simulink model "m20150807_motor28335_21"  (R2012b)
settings: Solver=FixedStepDiscrete  StartTime=0.0  StopTime=5  FixedStep=5e-5  RelTol=1e-3
PostLoadFcn:
  | c2000demoscallback(1);
  | Ts = 50e-6;
model workspace (MAT data in the model file):
  polePairs = 4
  encoderResolution = 2500
  indexOffset = 0
undefined symbols (not defined in the file or in its folder): Down, Up
libraries: c2833xlib x13, c28xdmclib x10, tiiqmathlib x8, simulink x4, c280xlib x4, idelinklib_common x4, c2000_demo_controls x1, idelinklib_tgtpref x1
settings Model: FPTRunName=Active  Creator=The MathWorks Inc.  LastModifiedBy=Krunal
settings DataIOCC: SignalLoggingSaveFormat=ModelDataLogs  SaveOutput=off  SaveTime=off
settings OptimizationCC: InlineParams=on  InlineInvariantSignals=on  InitFltsAndDblsToZero=on  NoFixptDivByZeroProtection=on  EfficientFloat2IntCast=on  EfficientMapNaN2IntZero=off  OptimizeModelRefInitCode=on
settings DebuggingCC: SignalResolutionControl=TryResolveAllWithWarning  InheritedTsInSrcMsg=none  MultiTaskDSMMsg=warning  MultiTaskCondExecSysMsg=none  SigSpecEnsureSampleTimeMsg=none  IntegerOverflowMsg=none  ParameterPrecisionLossMsg=none  FcnCallInpInsideContextMsg=UseLocalSettings  StrictBusMsg=None
settings HardwareCC: ProdBitPerChar=16  ProdBitPerInt=16  ProdBitPerPointer=16  ProdLargestAtomicInteger=Integer  ProdIntDivRoundTo=Zero  ProdEndianess=LittleEndian  ProdWordSize=16  ProdHWDeviceType=Texas Instruments->C2000  TargetBitPerChar=16  TargetBitPerInt=16  TargetBitPerPointer=16  TargetIntDivRoundTo=Zero  TargetEndianess=LittleEndian  TargetWordSize=16  TargetHWDeviceType=TI C2000
settings RTWCC: SystemTargetFile=idelink_ert.tlc  TLCOptions="-aCustomTestInterfaceFile=\"pil_gen_interface.tlc\""  GenerateMakefile=off  TemplateMakefile=none  Description=IDE Link ERT  ProcessScript=ccslink_ert_make_rtw_hook
settings CodeAppCC: IgnoreCustomStorageClasses=off
settings ConfigurationSet: Description=SimMechanics 2G

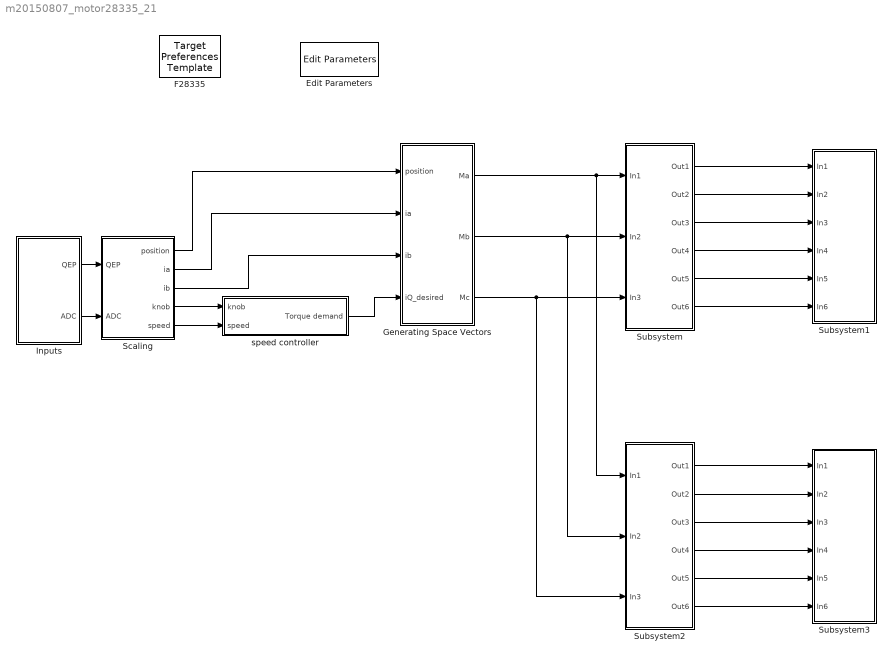
== system m20150807_motor28335_21 ==
  Edit Parameters : c2000_demo_controls/Edit Parameters  Priority=4  polePairs=4  encoderResolution=2500  IndexOffset=0
  F28335 : idelinklib_tgtpref/Target Preferences Template  Tag=ccslinktgtpref_ccsv5  library=off
  Generating Space Vectors : Subsystem
  Inputs : Subsystem
  Scaling : Subsystem
  Subsystem : Subsystem
  Subsystem1 : Subsystem
  Subsystem2 : Subsystem
  Subsystem3 : Subsystem
  speed controller : Subsystem
  wires:
  Scaling/1(position) -> Generating Space Vectors/1(position)
  Scaling/2(ia) -> Generating Space Vectors/2(ia)
  Scaling/3(ib) -> Generating Space Vectors/3(ib)
  Scaling/4(knob) -> speed controller/1(knob)
  Inputs/2(ADC) -> Scaling/2(ADC)
  speed controller/1(Torque demand) -> Generating Space Vectors/4(iQ_desired)
  Scaling/5(speed) -> speed controller/2(speed)
  Inputs/1(QEP) -> Scaling/1(QEP)
  Subsystem/1(Out1) -> Subsystem1/1(In1)
  Subsystem/2(Out2) -> Subsystem1/2(In2)
  Subsystem/3(Out3) -> Subsystem1/3(In3)
  Subsystem/4(Out4) -> Subsystem1/4(In4)
  Subsystem/5(Out5) -> Subsystem1/5(In5)
  Subsystem/6(Out6) -> Subsystem1/6(In6)
  Generating Space Vectors/1(Ma) -> Subsystem2/1(In1), Subsystem/1(In1)
  Generating Space Vectors/2(Mb) -> Subsystem2/2(In2), Subsystem/2(In2)
  Generating Space Vectors/3(Mc) -> Subsystem2/3(In3), Subsystem/3(In3)
  Subsystem2/1(Out1) -> Subsystem3/1(In1)
  Subsystem2/2(Out2) -> Subsystem3/2(In2)
  Subsystem2/3(Out3) -> Subsystem3/3(In3)
  Subsystem2/4(Out4) -> Subsystem3/4(In4)
  Subsystem2/5(Out5) -> Subsystem3/5(In5)
  Subsystem2/6(Out6) -> Subsystem3/6(In6)

== system m20150807_motor28335_21/Generating Space Vectors ==
  position : Inport
  ia : Inport  Port=2
  ib : Inport  Port=3
  iQ_desired : Inport  Port=4
  Generating Raw Space Vectors : Subsystem
  Rate Transition2 : RateTransition  Integrity=off
  Ma : Outport
  Mb : Outport  Port=2
  Mc : Outport  Port=3
  wires:
  ia/1 -> Generating Raw Space Vectors/1(Ia)
  ib/1 -> Generating Raw Space Vectors/2(Ib)
  position/1 -> Generating Raw Space Vectors/3(position)
  Generating Raw Space Vectors/1(Out1) -> Ma/1
  Generating Raw Space Vectors/2(Out2) -> Mb/1
  Generating Raw Space Vectors/3(Out3) -> Mc/1
  iQ_desired/1 -> Rate Transition2/1
  Rate Transition2/1 -> Generating Raw Space Vectors/4(iQ_desired)

== system m20150807_motor28335_21/Inputs ==
  note: Hardware Inputs
  ADC1 : c280xlib/ADC  useModule=A  useMode=Sequential  sourceSOC=Software  sourceSOC1=Software  sourceSOC2=ePWMxB  xint2_ADCSOC=31  Ts=Ts  dType=uint16  postInterrupt=off  numConversionsSingle=3  numConversionsDouble=1  conv0=ADCINA0  conv1=ADCINA1  conv2=ADCINA2  conv3=ADCINA3  conv4=ADCINA4  conv5=ADCINA5  conv6=ADCINA6  conv7=ADCINA7  conv8=ADCINB0  conv9=ADCINB1  conv10=ADCINB2  conv11=ADCINB3  conv12=ADCINB4  conv13=ADCINB5  conv14=ADCINB6  conv15=ADCINB7  convAB0=ADCINA0 and ADCINB0  convAB1=ADCINA1 and ADCINB1  convAB2=ADCINA2 and ADCINB2  convAB3=ADCINA3 and ADCINB3  convAB4=ADCINA4 and ADCINB4  convAB5=ADCINA5 and ADCINB5  convAB6=ADCINA6 and ADCINB6  convAB7=ADCINA7 and ADCINB7  convA0=ADCINA0  convA1=ADCINA1  convA2=ADCINA7  convA3=ADCINA3  convA4=ADCINA4  convA5=ADCINA5  convA6=ADCINA6  convA7=ADCINA7  convB0=ADCINB0  convB1=ADCINB1  convB2=ADCINB2  convB3=ADCINB3  convB4=ADCINB4  convB5=ADCINB5  convB6=ADCINB6  convB7=ADCINB7  c28xmultiPort=off  endma=off  chdma=1
  eQEP : c280xlib/eQEP  useModule=eQEP1  pcInputmode=Quadrature-count  externalClockrate=2x resolution: Count the rising/falling edge  swapPolarityselection=Clockwise  qdfOutputport=off  qapPolarityselection=off  qbpPolarityselection=off  qipPolarityselection=off  qspPolarityselection=off  igatePolarityselection=off  sampleTime=Ts  pcOutputport=on  pcMaximumvalue=65535  indexInitializationcheck=off  indexInitializationevent=Rising edge  strobeInitializationcheck=off  strobeInitializationevent=Rising edge  softwareInitializationcheck=off  softwareInitializationsource=Set to init value at start up  softwareInitializationmode=on  pcInitialvalue=2147483648  pcResetmode=Reset on an index event  ieloutputport=off  indexEventlatch=Rising edge  seloutputport=off  strobeEventlatch=Rising edge  pcefOutputport=off  enableEqepcapture=off  qctmrOutputport=off  qcprdOutputport=off  captureTimerprescaler=128  upEventprescaler=128  overflowErrorflag=off  directionErrorflag=off  captureTimerposition=On position counter read  unitTimerperiod=100000000  captureTimerlatch=off  capturePeriodlatch=off  positionCounterlatch=off  soenPolarityselection=off  spselPolarityselection=Index pin is used for sync output  compareValuesource=Specify via dialog  shadowMode=Load on QPOSCNT=0  compareValue=4294967295  syncOutputwidth=1  polaritySyncoutput=Active high  watchdogEnable=off  watchdogTimer=65535  outport1Datatype=auto  outport2Datatype=auto  outport3Datatype=auto  outport4Datatype=auto  outport5Datatype=auto  outport6Datatype=auto  outport7Datatype=auto  outport8Datatype=auto  outport9Datatype=auto  outport10Datatype=auto  outport11Datatype=auto  outport12Datatype=auto  eqepinterrupt_pce=off  eqepinterrupt_qpe=off  eqepinterrupt_qdc=off  eqepinterrupt_wto=off  eqepinterrupt_pcu=off  eqepinterrupt_pco=off  eqepinterrupt_pcr=off  eqepinterrupt_pcm=off  eqepinterrupt_sel=off  eqepinterrupt_iel=off  eqepinterrupt_uto=off  pheOutputport=off  watchdogOutputport=off  outport13Datatype=auto  outport14Datatype=auto
  QEP : Outport
  ADC : Outport  Port=2
  wires:
  eQEP/1 -> QEP/1
  ADC1/1 -> ADC/1

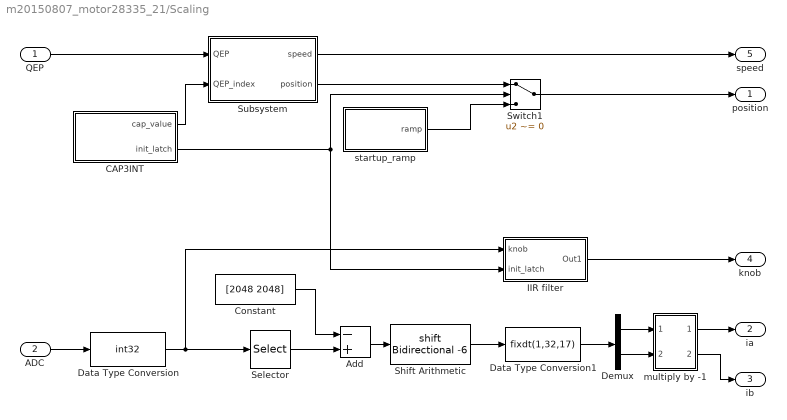
== system m20150807_motor28335_21/Scaling ==
  QEP : Inport
  ADC : Inport  Port=2
  Add : Sum  Inputs=-+
  CAP3INT : Subsystem
  Constant : Constant  Value=[2048 2048]  OutDataTypeStr=int32
  Data Type Conversion : DataTypeConversion  OutDataTypeStr=int32  ConvertRealWorld=Stored Integer (SI)
  Data Type Conversion1 : DataTypeConversion  OutDataTypeStr=fixdt(1,32,17)  ConvertRealWorld=Stored Integer (SI)
  Demux : Demux  Outputs=2
  IIR filter : Subsystem
  Selector : Selector  InputPortWidth=3  IndexOptions=Index vector (dialog)  Indices=[1 2]  OutputSizes=1
  Shift Arithmetic : ArithShift  BitShiftNumber=-6
  Subsystem : Subsystem
  Switch1 : Switch  Criteria=u2 ~= 0
  multiply by -1 : Subsystem
  startup_ramp : Subsystem
  position : Outport
  ia : Outport  Port=2
  ib : Outport  Port=3
  knob : Outport  Port=4
  speed : Outport  Port=5
  wires:
  CAP3INT/1(cap_value) -> Subsystem/2(QEP_index)
  CAP3INT/2(init_latch) -> Switch1/2, IIR filter/2(init_latch)
  startup_ramp/1(ramp) -> Switch1/3
  Subsystem/2(position) -> Switch1/1
  Data Type Conversion/1 -> Selector/1, IIR filter/1(knob)
  IIR filter/1(Out1) -> knob/1
  Constant/1 -> Add/1
  Selector/1 -> Add/2
  Add/1 -> Shift Arithmetic/1
  Shift Arithmetic/1 -> Data Type Conversion1/1
  Data Type Conversion1/1 -> Demux/1
  Demux/1 -> multiply by -1/1(In1)
  Demux/2 -> multiply by -1/2(In2)
  multiply by -1/1(Out1) -> ia/1
  multiply by -1/2(Out2) -> ib/1
  QEP/1 -> Subsystem/1(QEP)
  ADC/1 -> Data Type Conversion/1
  Switch1/1 -> position/1
  Subsystem/1(speed) -> speed/1

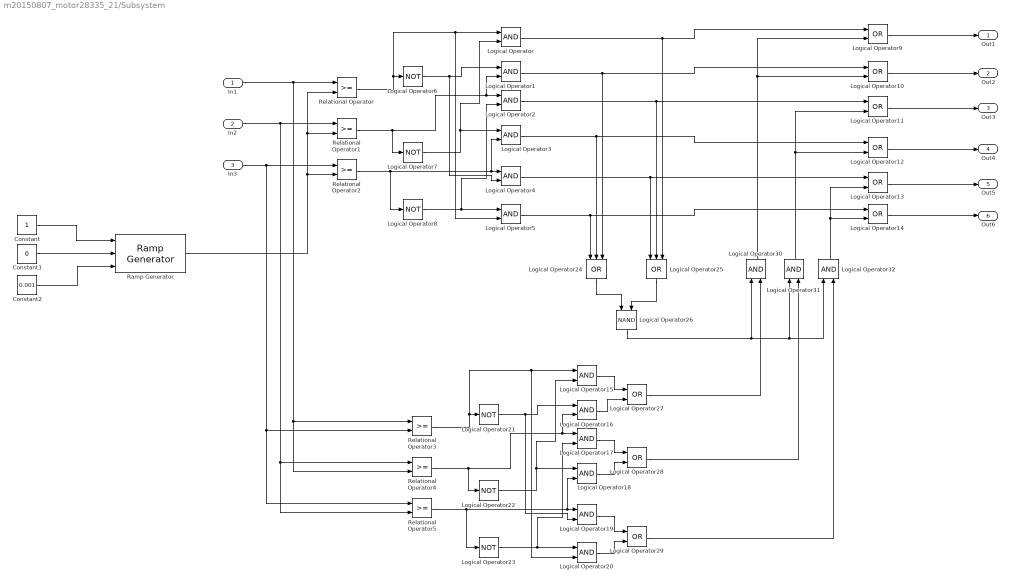
== system m20150807_motor28335_21/Subsystem ==
  In1 : Inport
  In2 : Inport  Port=2
  In3 : Inport  Port=3
  Constant : Constant  OutDataTypeStr=fixdt(1,32,2^-9,0)  SampleTime=0.001
  Constant1 : Constant  Value=0  OutDataTypeStr=fixdt(1,32,2^-9,0)
  Constant2 : Constant  Value=0.001  OutDataTypeStr=fixdt(1,32,2^-9,0)
  Logical Operator{,1..5,15..20,30..32} (15 alike) : Logic  AllPortsSameDT=off  OutDataTypeStr=boolean
  Logical Operator{9..14,27..29} (9 alike) : Logic  Operator=OR  AllPortsSameDT=off  OutDataTypeStr=boolean
  Logical Operator{6..8,21..23} (6 alike) : Logic  Operator=NOT  AllPortsSameDT=off  OutDataTypeStr=boolean
  Logical Operator24 : Logic  Operator=OR  Inputs=3  AllPortsSameDT=off  OutDataTypeStr=boolean
  Logical Operator25 : Logic  Operator=OR  Inputs=3  AllPortsSameDT=off  OutDataTypeStr=boolean
  Logical Operator26 : Logic  Operator=NAND  AllPortsSameDT=off  OutDataTypeStr=boolean
  Ramp Generator : c28xdmclib/Ramp Generator  step_angle_max=1
  Relational Operator{,1..5} (6 alike) : RelationalOperator  OutDataTypeStr=boolean
  Out1 : Outport
  Out2 : Outport  Port=2
  Out3 : Outport  Port=3
  Out4 : Outport  Port=4
  Out5 : Outport  Port=5
  Out6 : Outport  Port=6
  wires:
  Relational Operator2/1 -> Logical Operator8/1, Logical Operator3/2, Logical Operator4/1
  Relational Operator1/1 -> Logical Operator7/1, Logical Operator1/2, Logical Operator2/1
  Constant2/1 -> Ramp Generator/3
  Constant1/1 -> Ramp Generator/2
  Constant/1 -> Ramp Generator/1
  Relational Operator/1 -> Logical Operator6/1, Logical Operator5/2, Logical Operator/1
  Logical Operator6/1 -> Logical Operator4/2, Logical Operator1/1
  Logical Operator7/1 -> Logical Operator/2, Logical Operator3/1
  Logical Operator8/1 -> Logical Operator2/2, Logical Operator5/1
  Logical Operator14/1 -> Out6/1
  Logical Operator5/1 -> Logical Operator24/1, Logical Operator14/1
  Logical Operator13/1 -> Out5/1
  Logical Operator12/1 -> Out4/1
  Logical Operator11/1 -> Out3/1
  Logical Operator10/1 -> Out2/1
  Logical Operator9/1 -> Out1/1
  Logical Operator/1 -> Logical Operator9/1, Logical Operator25/3
  Logical Operator1/1 -> Logical Operator10/1, Logical Operator24/3
  Logical Operator2/1 -> Logical Operator25/2, Logical Operator11/1
  Logical Operator3/1 -> Logical Operator24/2, Logical Operator12/1
  Logical Operator4/1 -> Logical Operator25/1, Logical Operator13/1
  Relational Operator5/1 -> Logical Operator23/1, Logical Operator18/2, Logical Operator19/1
  Relational Operator4/1 -> Logical Operator22/1, Logical Operator16/2, Logical Operator17/1
  In2/1 -> Relational Operator5/2, Relational Operator4/1, Relational Operator1/1
  In1/1 -> Relational Operator4/2, Relational Operator3/1, Relational Operator/1
  In3/1 -> Relational Operator3/2, Relational Operator5/1, Relational Operator2/1
  Relational Operator3/1 -> Logical Operator21/1, Logical Operator20/2, Logical Operator15/1
  Logical Operator21/1 -> Logical Operator19/2, Logical Operator16/1
  Logical Operator22/1 -> Logical Operator15/2, Logical Operator18/1
  Logical Operator23/1 -> Logical Operator17/2, Logical Operator20/1
  Logical Operator20/1 -> Logical Operator29/2
  Logical Operator15/1 -> Logical Operator27/1
  Logical Operator16/1 -> Logical Operator27/2
  Logical Operator17/1 -> Logical Operator28/1
  Logical Operator18/1 -> Logical Operator28/2
  Logical Operator19/1 -> Logical Operator29/1
  Ramp Generator/1 -> Relational Operator2/2, Relational Operator1/2, Relational Operator/2
  Logical Operator24/1 -> Logical Operator26/1
  Logical Operator25/1 -> Logical Operator26/2
  Logical Operator26/1 -> Logical Operator30/1, Logical Operator31/1, Logical Operator32/1
  Logical Operator27/1 -> Logical Operator30/2
  Logical Operator28/1 -> Logical Operator31/2
  Logical Operator29/1 -> Logical Operator32/2
  Logical Operator30/1 -> Logical Operator10/2, Logical Operator9/2
  Logical Operator31/1 -> Logical Operator12/2, Logical Operator11/2
  Logical Operator32/1 -> Logical Operator14/2, Logical Operator13/2

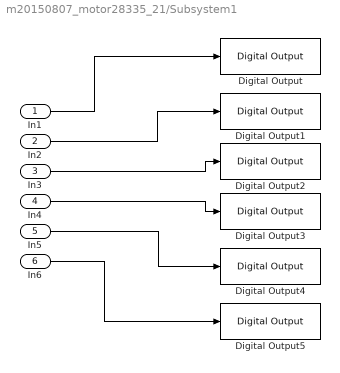
== system m20150807_motor28335_21/Subsystem1 ==
  In1 : Inport
  In2 : Inport  Port=2
  In3 : Inport  Port=3
  In4 : Inport  Port=4
  In5 : Inport  Port=5
  In6 : Inport  Port=6
  Digital Output : c2833xlib/Digital Output  GPIO_Number=GPIO0~GPIO7  GPIO_Bit0=on  GPIO_BIT0_Toggle=off  GPIO_Bit1=off  GPIO_BIT1_Toggle=off  GPIO_Bit2=off  GPIO_BIT2_Toggle=off  GPIO_Bit3=off  GPIO_BIT3_Toggle=off  GPIO_Bit4=off  GPIO_BIT4_Toggle=off  GPIO_Bit5=off  GPIO_BIT5_Toggle=off  GPIO_Bit6=off  GPIO_BIT6_Toggle=off  GPIO_Bit7=off  GPIO_BIT7_Toggle=off
  Digital Output1 : c2833xlib/Digital Output  GPIO_Number=GPIO0~GPIO7  GPIO_Bit0=off  GPIO_BIT0_Toggle=off  GPIO_Bit1=on  GPIO_BIT1_Toggle=off  GPIO_Bit2=off  GPIO_BIT2_Toggle=off  GPIO_Bit3=off  GPIO_BIT3_Toggle=off  GPIO_Bit4=off  GPIO_BIT4_Toggle=off  GPIO_Bit5=off  GPIO_BIT5_Toggle=off  GPIO_Bit6=off  GPIO_BIT6_Toggle=off  GPIO_Bit7=off  GPIO_BIT7_Toggle=off
  Digital Output2 : c2833xlib/Digital Output  GPIO_Number=GPIO0~GPIO7  GPIO_Bit0=off  GPIO_BIT0_Toggle=off  GPIO_Bit1=off  GPIO_BIT1_Toggle=off  GPIO_Bit2=on  GPIO_BIT2_Toggle=off  GPIO_Bit3=off  GPIO_BIT3_Toggle=off  GPIO_Bit4=off  GPIO_BIT4_Toggle=off  GPIO_Bit5=off  GPIO_BIT5_Toggle=off  GPIO_Bit6=off  GPIO_BIT6_Toggle=off  GPIO_Bit7=off  GPIO_BIT7_Toggle=off
  Digital Output3 : c2833xlib/Digital Output  GPIO_Number=GPIO0~GPIO7  GPIO_Bit0=off  GPIO_BIT0_Toggle=off  GPIO_Bit1=off  GPIO_BIT1_Toggle=off  GPIO_Bit2=off  GPIO_BIT2_Toggle=off  GPIO_Bit3=on  GPIO_BIT3_Toggle=off  GPIO_Bit4=off  GPIO_BIT4_Toggle=off  GPIO_Bit5=off  GPIO_BIT5_Toggle=off  GPIO_Bit6=off  GPIO_BIT6_Toggle=off  GPIO_Bit7=off  GPIO_BIT7_Toggle=off
  Digital Output4 : c2833xlib/Digital Output  GPIO_Number=GPIO0~GPIO7  GPIO_Bit0=off  GPIO_BIT0_Toggle=off  GPIO_Bit1=off  GPIO_BIT1_Toggle=off  GPIO_Bit2=off  GPIO_BIT2_Toggle=off  GPIO_Bit3=off  GPIO_BIT3_Toggle=off  GPIO_Bit4=on  GPIO_BIT4_Toggle=off  GPIO_Bit5=off  GPIO_BIT5_Toggle=off  GPIO_Bit6=off  GPIO_BIT6_Toggle=off  GPIO_Bit7=off  GPIO_BIT7_Toggle=off
  Digital Output5 : c2833xlib/Digital Output  GPIO_Number=GPIO0~GPIO7  GPIO_Bit0=off  GPIO_BIT0_Toggle=off  GPIO_Bit1=off  GPIO_BIT1_Toggle=off  GPIO_Bit2=off  GPIO_BIT2_Toggle=off  GPIO_Bit3=off  GPIO_BIT3_Toggle=off  GPIO_Bit4=off  GPIO_BIT4_Toggle=off  GPIO_Bit5=on  GPIO_BIT5_Toggle=off  GPIO_Bit6=off  GPIO_BIT6_Toggle=off  GPIO_Bit7=off  GPIO_BIT7_Toggle=off
  wires:
  In6/1 -> Digital Output5/1
  In1/1 -> Digital Output/1
  In5/1 -> Digital Output4/1
  In4/1 -> Digital Output3/1
  In3/1 -> Digital Output2/1
  In2/1 -> Digital Output1/1

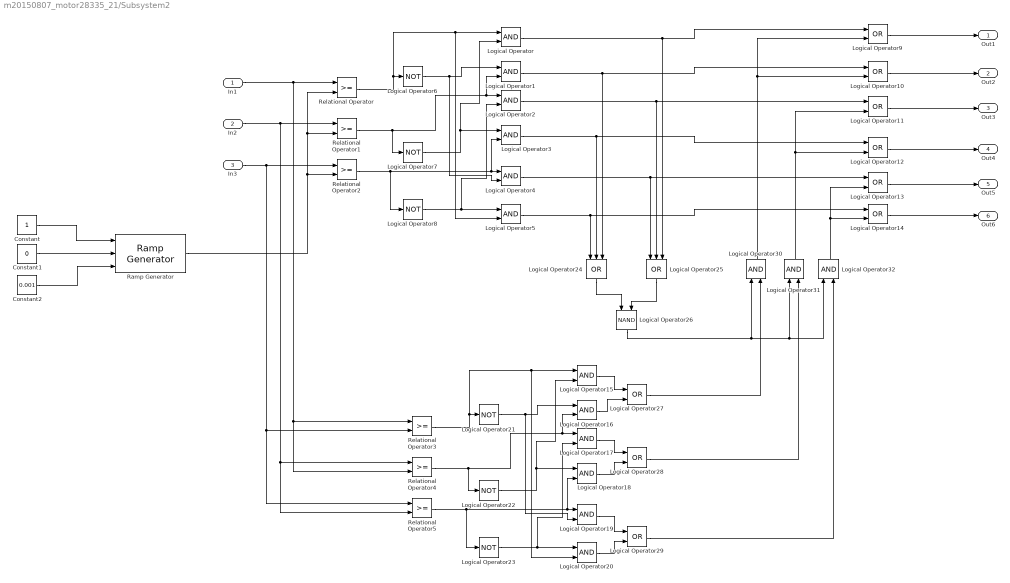
== system m20150807_motor28335_21/Subsystem2 ==
  In1 : Inport
  In2 : Inport  Port=2
  In3 : Inport  Port=3
  Constant : Constant  OutDataTypeStr=fixdt(1,32,2^-9,0)  SampleTime=0.001
  Constant1 : Constant  Value=0  OutDataTypeStr=fixdt(1,32,2^-9,0)
  Constant2 : Constant  Value=0.001  OutDataTypeStr=fixdt(1,32,2^-9,0)
  Logical Operator{,1..5,15..20,30..32} (15 alike) : Logic  AllPortsSameDT=off  OutDataTypeStr=boolean
  Logical Operator{9..14,27..29} (9 alike) : Logic  Operator=OR  AllPortsSameDT=off  OutDataTypeStr=boolean
  Logical Operator{6..8,21..23} (6 alike) : Logic  Operator=NOT  AllPortsSameDT=off  OutDataTypeStr=boolean
  Logical Operator24 : Logic  Operator=OR  Inputs=3  AllPortsSameDT=off  OutDataTypeStr=boolean
  Logical Operator25 : Logic  Operator=OR  Inputs=3  AllPortsSameDT=off  OutDataTypeStr=boolean
  Logical Operator26 : Logic  Operator=NAND  AllPortsSameDT=off  OutDataTypeStr=boolean
  Ramp Generator : c28xdmclib/Ramp Generator  step_angle_max=1
  Relational Operator{,1..5} (6 alike) : RelationalOperator  OutDataTypeStr=boolean
  Out1 : Outport
  Out2 : Outport  Port=2
  Out3 : Outport  Port=3
  Out4 : Outport  Port=4
  Out5 : Outport  Port=5
  Out6 : Outport  Port=6
  wires:
  Relational Operator2/1 -> Logical Operator8/1, Logical Operator3/2, Logical Operator4/1
  Relational Operator1/1 -> Logical Operator7/1, Logical Operator1/2, Logical Operator2/1
  Constant2/1 -> Ramp Generator/3
  Constant1/1 -> Ramp Generator/2
  Constant/1 -> Ramp Generator/1
  Relational Operator/1 -> Logical Operator6/1, Logical Operator5/2, Logical Operator/1
  Logical Operator6/1 -> Logical Operator4/2, Logical Operator1/1
  Logical Operator7/1 -> Logical Operator/2, Logical Operator3/1
  Logical Operator8/1 -> Logical Operator2/2, Logical Operator5/1
  Logical Operator14/1 -> Out6/1
  Logical Operator5/1 -> Logical Operator24/1, Logical Operator14/1
  Logical Operator13/1 -> Out5/1
  Logical Operator12/1 -> Out4/1
  Logical Operator11/1 -> Out3/1
  Logical Operator10/1 -> Out2/1
  Logical Operator9/1 -> Out1/1
  Logical Operator/1 -> Logical Operator9/1, Logical Operator25/3
  Logical Operator1/1 -> Logical Operator10/1, Logical Operator24/3
  Logical Operator2/1 -> Logical Operator25/2, Logical Operator11/1
  Logical Operator3/1 -> Logical Operator24/2, Logical Operator12/1
  Logical Operator4/1 -> Logical Operator25/1, Logical Operator13/1
  Relational Operator5/1 -> Logical Operator23/1, Logical Operator18/2, Logical Operator19/1
  Relational Operator4/1 -> Logical Operator22/1, Logical Operator16/2, Logical Operator17/1
  In2/1 -> Relational Operator5/2, Relational Operator4/1, Relational Operator1/1
  In1/1 -> Relational Operator4/2, Relational Operator3/1, Relational Operator/1
  In3/1 -> Relational Operator3/2, Relational Operator5/1, Relational Operator2/1
  Relational Operator3/1 -> Logical Operator21/1, Logical Operator20/2, Logical Operator15/1
  Logical Operator21/1 -> Logical Operator19/2, Logical Operator16/1
  Logical Operator22/1 -> Logical Operator15/2, Logical Operator18/1
  Logical Operator23/1 -> Logical Operator17/2, Logical Operator20/1
  Logical Operator20/1 -> Logical Operator29/2
  Logical Operator15/1 -> Logical Operator27/1
  Logical Operator16/1 -> Logical Operator27/2
  Logical Operator17/1 -> Logical Operator28/1
  Logical Operator18/1 -> Logical Operator28/2
  Logical Operator19/1 -> Logical Operator29/1
  Ramp Generator/1 -> Relational Operator2/2, Relational Operator1/2, Relational Operator/2
  Logical Operator24/1 -> Logical Operator26/1
  Logical Operator25/1 -> Logical Operator26/2
  Logical Operator26/1 -> Logical Operator30/1, Logical Operator31/1, Logical Operator32/1
  Logical Operator27/1 -> Logical Operator30/2
  Logical Operator28/1 -> Logical Operator31/2
  Logical Operator29/1 -> Logical Operator32/2
  Logical Operator30/1 -> Logical Operator10/2, Logical Operator9/2
  Logical Operator31/1 -> Logical Operator12/2, Logical Operator11/2
  Logical Operator32/1 -> Logical Operator14/2, Logical Operator13/2

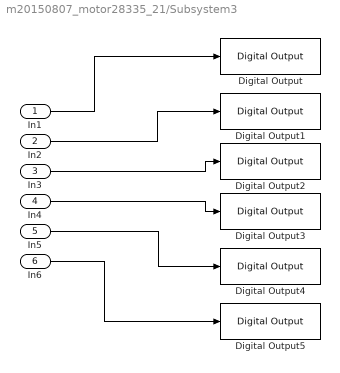
== system m20150807_motor28335_21/Subsystem3 ==
  In1 : Inport
  In2 : Inport  Port=2
  In3 : Inport  Port=3
  In4 : Inport  Port=4
  In5 : Inport  Port=5
  In6 : Inport  Port=6
  Digital Output : c2833xlib/Digital Output  GPIO_Number=GPIO8~GPIO15  GPIO_Bit0=on  GPIO_BIT0_Toggle=off  GPIO_Bit1=off  GPIO_BIT1_Toggle=off  GPIO_Bit2=off  GPIO_BIT2_Toggle=off  GPIO_Bit3=off  GPIO_BIT3_Toggle=off  GPIO_Bit4=off  GPIO_BIT4_Toggle=off  GPIO_Bit5=off  GPIO_BIT5_Toggle=off  GPIO_Bit6=off  GPIO_BIT6_Toggle=off  GPIO_Bit7=off  GPIO_BIT7_Toggle=off
  Digital Output1 : c2833xlib/Digital Output  GPIO_Number=GPIO8~GPIO15  GPIO_Bit0=off  GPIO_BIT0_Toggle=off  GPIO_Bit1=on  GPIO_BIT1_Toggle=off  GPIO_Bit2=off  GPIO_BIT2_Toggle=off  GPIO_Bit3=off  GPIO_BIT3_Toggle=off  GPIO_Bit4=off  GPIO_BIT4_Toggle=off  GPIO_Bit5=off  GPIO_BIT5_Toggle=off  GPIO_Bit6=off  GPIO_BIT6_Toggle=off  GPIO_Bit7=off  GPIO_BIT7_Toggle=off
  Digital Output2 : c2833xlib/Digital Output  GPIO_Number=GPIO8~GPIO15  GPIO_Bit0=off  GPIO_BIT0_Toggle=off  GPIO_Bit1=off  GPIO_BIT1_Toggle=off  GPIO_Bit2=on  GPIO_BIT2_Toggle=off  GPIO_Bit3=off  GPIO_BIT3_Toggle=off  GPIO_Bit4=off  GPIO_BIT4_Toggle=off  GPIO_Bit5=off  GPIO_BIT5_Toggle=off  GPIO_Bit6=off  GPIO_BIT6_Toggle=off  GPIO_Bit7=off  GPIO_BIT7_Toggle=off
  Digital Output3 : c2833xlib/Digital Output  GPIO_Number=GPIO8~GPIO15  GPIO_Bit0=off  GPIO_BIT0_Toggle=off  GPIO_Bit1=off  GPIO_BIT1_Toggle=off  GPIO_Bit2=off  GPIO_BIT2_Toggle=off  GPIO_Bit3=on  GPIO_BIT3_Toggle=off  GPIO_Bit4=off  GPIO_BIT4_Toggle=off  GPIO_Bit5=off  GPIO_BIT5_Toggle=off  GPIO_Bit6=off  GPIO_BIT6_Toggle=off  GPIO_Bit7=off  GPIO_BIT7_Toggle=off
  Digital Output4 : c2833xlib/Digital Output  GPIO_Number=GPIO8~GPIO15  GPIO_Bit0=off  GPIO_BIT0_Toggle=off  GPIO_Bit1=off  GPIO_BIT1_Toggle=off  GPIO_Bit2=off  GPIO_BIT2_Toggle=off  GPIO_Bit3=off  GPIO_BIT3_Toggle=off  GPIO_Bit4=on  GPIO_BIT4_Toggle=off  GPIO_Bit5=off  GPIO_BIT5_Toggle=off  GPIO_Bit6=off  GPIO_BIT6_Toggle=off  GPIO_Bit7=off  GPIO_BIT7_Toggle=off
  Digital Output5 : c2833xlib/Digital Output  GPIO_Number=GPIO0~GPIO7  GPIO_Bit0=off  GPIO_BIT0_Toggle=off  GPIO_Bit1=off  GPIO_BIT1_Toggle=off  GPIO_Bit2=off  GPIO_BIT2_Toggle=off  GPIO_Bit3=off  GPIO_BIT3_Toggle=off  GPIO_Bit4=off  GPIO_BIT4_Toggle=off  GPIO_Bit5=on  GPIO_BIT5_Toggle=off  GPIO_Bit6=off  GPIO_BIT6_Toggle=off  GPIO_Bit7=off  GPIO_BIT7_Toggle=off
  wires:
  In6/1 -> Digital Output5/1
  In1/1 -> Digital Output/1
  In5/1 -> Digital Output4/1
  In4/1 -> Digital Output3/1
  In3/1 -> Digital Output2/1
  In2/1 -> Digital Output1/1

== system m20150807_motor28335_21/speed controller ==
  knob : Inport
  speed : Inport  Port=2
  PID Controller : c28xdmclib/PID Controller  proportionalGain=0.5  integralGain=0.1  correctionGain=0.1  derivativeGain=0  minOutput=-1  maxOutput=1
  Speed Controller : Scope  NumInputPorts=3
      settings: TimeRange=5  YMin=-0.1~0~0  YMax=0.1~0.5055386726791493~0.5321400000000003
  Torque demand : Outport
  wires:
  PID Controller/1 -> Torque demand/1, Speed Controller/1  "Torque demand"
  speed/1 -> PID Controller/2, Speed Controller/3  "Actual speed"
  knob/1 -> PID Controller/1, Speed Controller/2  "Desired speed"

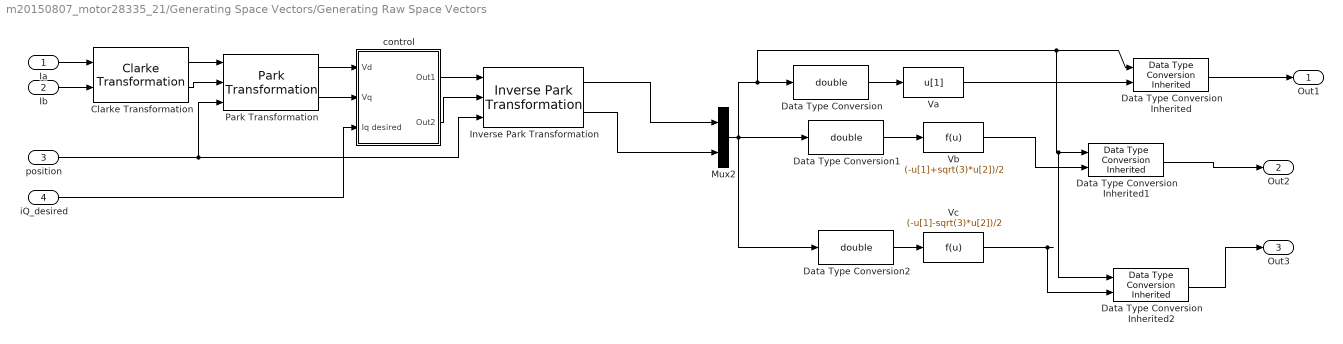
== system m20150807_motor28335_21/Generating Space Vectors/Generating Raw Space Vectors ==
  Ia : Inport
  Ib : Inport  Port=2
  position : Inport  Port=3
  iQ_desired : Inport  Port=4
  Clarke Transformation : c28xdmclib/Clarke Transformation
  Data Type Conversion Inherited : simulink/Signal Attributes/Data Type Conversion Inherited  ConvertRealWorld=Real World Value  DoSatur=off
  Data Type Conversion Inherited1 : simulink/Signal Attributes/Data Type Conversion Inherited  ConvertRealWorld=Real World Value  DoSatur=off
  Data Type Conversion Inherited2 : simulink/Signal Attributes/Data Type Conversion Inherited  ConvertRealWorld=Real World Value  DoSatur=off
  Data Type Conversion : DataTypeConversion  OutDataTypeStr=double
  Data Type Conversion1 : DataTypeConversion  OutDataTypeStr=double
  Data Type Conversion2 : DataTypeConversion  OutDataTypeStr=double
  Inverse Park Transformation : c28xdmclib/Inverse Park Transformation
  Mux2 : Mux  Inputs=2
  Park Transformation : c28xdmclib/Park Transformation
  Va : Fcn  Expr=u[1]
  Vb : Fcn  Expr=(-u[1]+sqrt(3)*u[2])/2
  Vc : Fcn  Expr=(-u[1]-sqrt(3)*u[2])/2
  control : Subsystem
  Out1 : Outport
  Out2 : Outport  Port=2
  Out3 : Outport  Port=3
  wires:
  Vb/1 -> Data Type Conversion Inherited1/2
  position/1 -> Park Transformation/3, Inverse Park Transformation/3
  Vc/1 -> Data Type Conversion Inherited2/2
  Ia/1 -> Clarke Transformation/1
  Ib/1 -> Clarke Transformation/2
  Clarke Transformation/1 -> Park Transformation/1
  Clarke Transformation/2 -> Park Transformation/2
  iQ_desired/1 -> control/3(Iq desired)
  Park Transformation/1 -> control/1(Vd)
  Park Transformation/2 -> control/2(Vq)
  control/1(Out1) -> Inverse Park Transformation/1
  control/2(Out2) -> Inverse Park Transformation/2
  Inverse Park Transformation/1 -> Mux2/1
  Inverse Park Transformation/2 -> Mux2/2
  Data Type Conversion/1 -> Va/1
  Data Type Conversion1/1 -> Vb/1
  Data Type Conversion2/1 -> Vc/1
  Data Type Conversion Inherited/1 -> Out1/1
  Data Type Conversion Inherited1/1 -> Out2/1
  Data Type Conversion Inherited2/1 -> Out3/1
  Va/1 -> Data Type Conversion Inherited/2
  Mux2/1 -> Data Type Conversion1/1, Data Type Conversion Inherited2/1, Data Type Conversion Inherited1/1, Data Type Conversion Inherited/1, Data Type Conversion/1, Data Type Conversion2/1

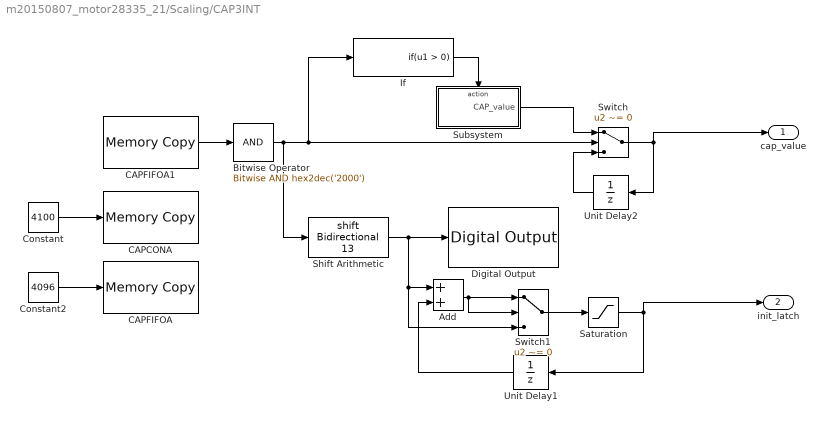
== system m20150807_motor28335_21/Scaling/CAP3INT ==
  Add : Sum  OutDataTypeStr=uint16
  Bitwise Operator : simulink/Logic and Bit Operations/Bitwise Operator  logicop=AND  UseBitMask=on  BitMask=hex2dec('2000')  BitMaskRealWorld=Stored Integer
  CAPCONA : idelinklib_common/Memory Copy  copyFrom=Input port  copyFromAddressSource=Specify via dialog  copyFromAddress=hex2dec('00001000')  copyFromSrcCode=myVariableSrc  dataTypeFrom=uint16  dataDimensionFrom=1  useOffsetFrom=off  offsetFromSrc=Specify via dialog  offsetFrom=0  strideFrom=1  copyTo=Specified address  copyToAddressSource=Specify via dialog  copyToAddress=hex2dec('7420')  copyToSrcCode=myVariableDst  dataTypeTo=uint16  useOffsetTo=off  offsetToSrc=Specify via dialog  offsetTo=0  strideTo=1  sampleTime=inf  useInitValue=on  initValueSrc=Specify constant value  initValue=hex2dec('1004')  initValueSrcCode=myInitValueVariable  useAsMask=off  maskOperator=bitwise AND  useTermValue=off  termValue=1  isRealtimeEnabled=off  emitCCBeforeWrite=off  CCBeforeWrite=/* Custom Code Before Write*/  emitCCAfterWrite=off  CCAfterWrite=/* Custom Code After Write*/  useDMACopy=off  enableBlockingMode=off
  CAPFIFOA : idelinklib_common/Memory Copy  copyFrom=Input port  copyFromAddressSource=Specify via dialog  copyFromAddress=hex2dec('00001000')  copyFromSrcCode=myVariableSrc  dataTypeFrom=uint16  dataDimensionFrom=1  useOffsetFrom=off  offsetFromSrc=Specify via dialog  offsetFrom=0  strideFrom=1  copyTo=Specified address  copyToAddressSource=Specify via dialog  copyToAddress=hex2dec('7422')  copyToSrcCode=myVariableDst  dataTypeTo=uint16  useOffsetTo=off  offsetToSrc=Specify via dialog  offsetTo=0  strideTo=1  sampleTime=inf  useInitValue=on  initValueSrc=Specify constant value  initValue=hex2dec('1000')  initValueSrcCode=myInitValueVariable  useAsMask=off  maskOperator=bitwise AND  useTermValue=off  termValue=1  isRealtimeEnabled=off  emitCCBeforeWrite=off  CCBeforeWrite=/* Custom Code Before Write*/  emitCCAfterWrite=off  CCAfterWrite=/* Custom Code After Write*/  useDMACopy=off  enableBlockingMode=off
  CAPFIFOA1 : idelinklib_common/Memory Copy  copyFrom=Specified address  copyFromAddressSource=Specify via dialog  copyFromAddress=hex2dec('7422')  copyFromSrcCode=myVariableSrc  dataTypeFrom=uint16  dataDimensionFrom=1  useOffsetFrom=off  offsetFromSrc=Specify via dialog  offsetFrom=0  strideFrom=1  copyTo=Output port  copyToAddressSource=Specify via dialog  copyToAddress=hex2dec('00002000')  copyToSrcCode=myVariableDst  dataTypeTo=uint16  useOffsetTo=off  offsetToSrc=Specify via dialog  offsetTo=0  strideTo=1  sampleTime=-1  useInitValue=off  initValueSrc=Specify constant value  initValue=1  initValueSrcCode=myInitValueVariable  useAsMask=off  maskOperator=bitwise AND  useTermValue=off  termValue=1  isRealtimeEnabled=off  emitCCBeforeWrite=off  CCBeforeWrite=/* Custom Code Before Write*/  emitCCAfterWrite=off  CCAfterWrite=/* Custom Code After Write*/  useDMACopy=off  enableBlockingMode=off
  Constant : Constant  Value=4100  OutDataTypeStr=uint16
  Constant2 : Constant  Value=4096  OutDataTypeStr=uint16
  Digital Output : c2833xlib/Digital Output  GPIO_Number=GPIO32~GPIO39  GPIO_Bit0=on  GPIO_BIT0_Toggle=off  GPIO_Bit1=off  GPIO_BIT1_Toggle=off  GPIO_Bit2=off  GPIO_BIT2_Toggle=off  GPIO_Bit3=off  GPIO_BIT3_Toggle=off  GPIO_Bit4=off  GPIO_BIT4_Toggle=off  GPIO_Bit5=off  GPIO_BIT5_Toggle=off  GPIO_Bit6=off  GPIO_BIT6_Toggle=off  GPIO_Bit7=off  GPIO_BIT7_Toggle=off
  If : If  ShowElse=off
  Saturation : Saturate  UpperLimit=1  LowerLimit=0
  Shift Arithmetic : ArithShift  BitShiftNumber=13
  Subsystem : Subsystem  TreatAsAtomicUnit=on
  Switch : Switch  Criteria=u2 ~= 0
  Switch1 : Switch  Criteria=u2 ~= 0  InputSameDT=on
  Unit Delay1 : UnitDelay  SampleTime=-1
  Unit Delay2 : UnitDelay  SampleTime=-1
  cap_value : Outport
  init_latch : Outport  Port=2
  wires:
  CAPFIFOA1/1 -> Bitwise Operator/1
  Subsystem/1(CAP_value) -> Switch/1
  Unit Delay2/1 -> Switch/3
  If/1 -> Subsystem/Action
  Bitwise Operator/1 -> If/1, Switch/2, Shift Arithmetic/1
  Shift Arithmetic/1 -> Digital Output/1, Add/1, Switch1/3
  Unit Delay1/1 -> Add/2
  Add/1 -> Switch1/2, Switch1/1
  Switch1/1 -> Saturation/1
  Switch/1 -> cap_value/1, Unit Delay2/1
  Saturation/1 -> init_latch/1, Unit Delay1/1
  Constant/1 -> CAPCONA/1
  Constant2/1 -> CAPFIFOA/1

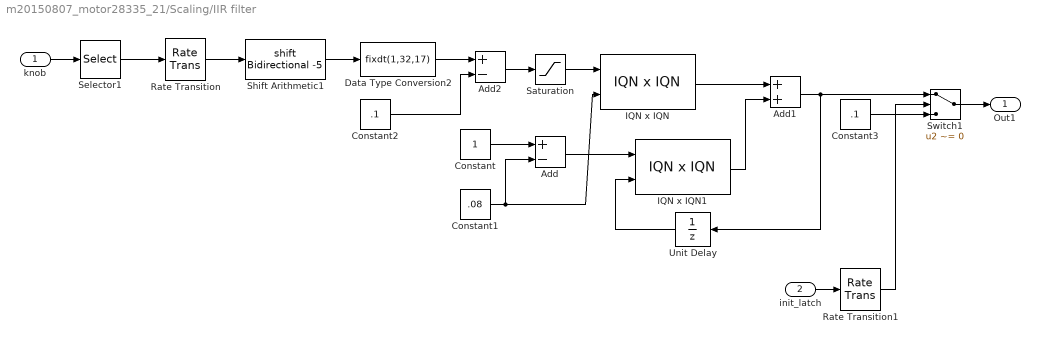
== system m20150807_motor28335_21/Scaling/IIR filter ==
  knob : Inport
  init_latch : Inport  Port=2
  Add : Sum  Inputs=+-
  Add1 : Sum
  Add2 : Sum  Inputs=+-
  Constant : Constant  OutDataTypeStr=fixdt(1,32,17)
  Constant1 : Constant  Value=.08  OutDataTypeStr=fixdt(1,32,17)
  Constant2 : Constant  Value=.1  OutDataTypeStr=fixdt(1,32,17)
  Constant3 : Constant  Value=.1  OutDataTypeStr=fixdt(1,32,17)
  Data Type Conversion2 : DataTypeConversion  OutDataTypeStr=fixdt(1,32,17)  ConvertRealWorld=Stored Integer (SI)
  IQN x IQN : tiiqmathlib/IQN x IQN  multiplyOption=Multiply
  IQN x IQN1 : tiiqmathlib/IQN x IQN  multiplyOption=Multiply
  Rate Transition : RateTransition  Integrity=off  OutPortSampleTime=0.01
  Rate Transition1 : RateTransition  Integrity=off  OutPortSampleTime=0.01
  Saturation : Saturate  UpperLimit=1  LowerLimit=0
  Selector1 : Selector  InputPortWidth=3  IndexOptions=Index vector (dialog)  Indices=[3]  OutputSizes=1
  Shift Arithmetic1 : ArithShift  BitShiftNumber=-5
  Switch1 : Switch  Criteria=u2 ~= 0
  Unit Delay : UnitDelay  SampleTime=-1
  Out1 : Outport
  wires:
  Selector1/1 -> Rate Transition/1
  knob/1 -> Selector1/1
  Constant/1 -> Add/1
  Constant1/1 -> Add/2, IQN x IQN/2
  IQN x IQN/1 -> Add1/1
  Add/1 -> IQN x IQN1/1
  Add1/1 -> Unit Delay/1, Switch1/1
  Unit Delay/1 -> IQN x IQN1/2
  IQN x IQN1/1 -> Add1/2
  Shift Arithmetic1/1 -> Data Type Conversion2/1
  Constant2/1 -> Add2/2
  Data Type Conversion2/1 -> Add2/1
  Add2/1 -> Saturation/1
  init_latch/1 -> Rate Transition1/1
  Constant3/1 -> Switch1/3
  Switch1/1 -> Out1/1
  Rate Transition1/1 -> Switch1/2
  Rate Transition/1 -> Shift Arithmetic1/1
  Saturation/1 -> IQN x IQN/1

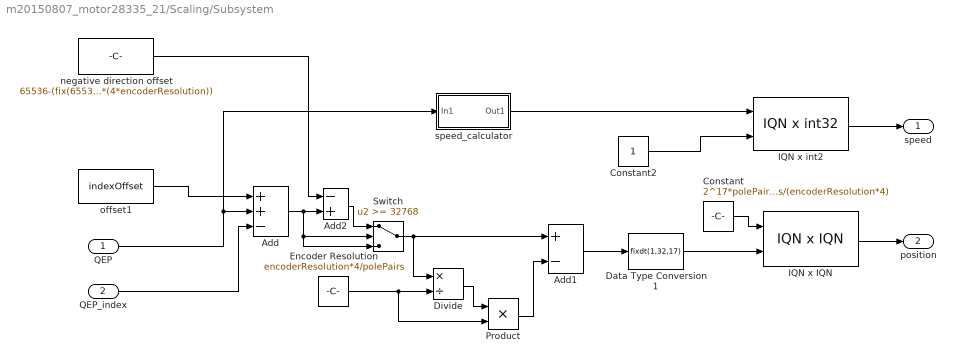
== system m20150807_motor28335_21/Scaling/Subsystem ==
  QEP : Inport
  QEP_index : Inport  Port=2
  Add : Sum  Inputs=++-  OutDataTypeStr=Inherit: Same as first input
  Add1 : Sum  Inputs=+-  OutDataTypeStr=uint16  RndMeth=Nearest
  Add2 : Sum  Inputs=-+  OutDataTypeStr=Inherit: Same as first input
  Constant : Constant  Value=2^17*polePairs/(encoderResolution*4)  OutDataTypeStr=fixdt(1,32,17)
  Constant2 : Constant  OutDataTypeStr=int32
  Data Type Conversion1 : DataTypeConversion  OutDataTypeStr=fixdt(1,32,17)  ConvertRealWorld=Stored Integer (SI)
  Divide : Product  Inputs=*/  OutDataTypeStr=uint16
  Encoder Resolution : Constant  Value=encoderResolution*4/polePairs  OutDataTypeStr=uint16
  IQN x IQN : tiiqmathlib/IQN x IQN  multiplyOption=Multiply
  IQN x int2 : tiiqmathlib/IQN x int32
  Product : Product  OutDataTypeStr=uint16  RndMeth=Zero
  Switch : Switch  Threshold=32768
  negative direction offset : Constant  Value=65536-(fix(65536/(4*encoderResolution))*(4*encoderResolution))  OutDataTypeStr=uint16
  offset1 : Constant  Value=indexOffset  OutDataTypeStr=uint16
  speed_calculator : Subsystem
  speed : Outport
  position : Outport  Port=2
  wires:
  Add/1 -> Switch/3, Switch/2, Add2/2
  Encoder Resolution/1 -> Product/2, Divide/2
  Divide/1 -> Product/1
  Product/1 -> Add1/2
  negative direction offset/1 -> Add2/1
  Add2/1 -> Switch/1
  Switch/1 -> Divide/1, Add1/1
  QEP/1 -> Add/2, speed_calculator/1(In1)
  QEP_index/1 -> Add/3
  Add1/1 -> Data Type Conversion1/1
  offset1/1 -> Add/1
  Constant2/1 -> IQN x int2/2
  IQN x int2/1 -> speed/1
  speed_calculator/1(Out1) -> IQN x int2/1
  Constant/1 -> IQN x IQN/1
  Data Type Conversion1/1 -> IQN x IQN/2
  IQN x IQN/1 -> position/1

== system m20150807_motor28335_21/Scaling/multiply by -1 ==
  In1 : Inport
  In2 : Inport  Port=2
  Constant1 : Constant  Value=-1  OutDataTypeStr=int32
  Constant3 : Constant  Value=-1  OutDataTypeStr=int32
  IQN x int1 : tiiqmathlib/IQN x int32
  IQN x int2 : tiiqmathlib/IQN x int32
  Out1 : Outport
  Out2 : Outport  Port=2
  wires:
  Constant3/1 -> IQN x int1/2
  In1/1 -> IQN x int1/1
  IQN x int1/1 -> Out1/1
  Constant1/1 -> IQN x int2/2
  In2/1 -> IQN x int2/1
  IQN x int2/1 -> Out2/1

== system m20150807_motor28335_21/Scaling/startup_ramp ==
  Ramp Control : c28xdmclib/Ramp Control  rmp_dly_max=1  rmp_lo_limit=0  rmp_hi_limit=1
  Ramp Generator : c28xdmclib/Ramp Generator  step_angle_max=0.005
  Terminator : Terminator
  offset : Constant  Value=0.1  OutDataTypeStr=fixdt(1,32,17)  SampleTime=-1
  offset1 : Constant  OutDataTypeStr=fixdt(1,32,17)  SampleTime=-1
  offset2 : Constant  Value=0  OutDataTypeStr=fixdt(1,32,17)  SampleTime=-1
  ramp : Outport
  wires:
  Ramp Control/1 -> Ramp Generator/3
  offset/1 -> Ramp Control/1
  Ramp Control/2 -> Terminator/1
  offset2/1 -> Ramp Generator/2
  offset1/1 -> Ramp Generator/1
  Ramp Generator/1 -> ramp/1

== system m20150807_motor28335_21/Generating Space Vectors/Generating Raw Space Vectors/control ==
  Vd : Inport
  Vq : Inport  Port=2
  Iq desired : Inport  Port=3
  Constant1 : Constant  Value=0  OutDataTypeStr=fixdt(1,32,17)
  PID Controller : c28xdmclib/PID Controller  proportionalGain=0.2  integralGain=0.002  correctionGain=0.002  derivativeGain=0  minOutput=-1  maxOutput=1
  PID Controller1 : c28xdmclib/PID Controller  proportionalGain=0.2  integralGain=0.002  correctionGain=0.002  derivativeGain=0  minOutput=-1  maxOutput=1
  saturation : Subsystem
  Out1 : Outport
  Out2 : Outport  Port=2
  wires:
  Vd/1 -> PID Controller/2
  Vq/1 -> PID Controller1/2
  PID Controller/1 -> saturation/1(In1)
  saturation/1(Out1) -> Out1/1
  saturation/2(Out2) -> Out2/1
  Constant1/1 -> PID Controller/1
  PID Controller1/1 -> saturation/2(In2)
  Iq desired/1 -> PID Controller1/1

== system m20150807_motor28335_21/Scaling/CAP3INT/Subsystem ==
  Action Port : ActionPort  PropagateVarSize=During execution  ActionType=then
  CAP1FBOT : idelinklib_common/Memory Copy  copyFrom=Specified address  copyFromAddressSource=Specify via dialog  copyFromAddress=hex2dec('7429')  copyFromSrcCode=myVariableSrc  dataTypeFrom=uint16  dataDimensionFrom=1  useOffsetFrom=off  offsetFromSrc=Specify via dialog  offsetFrom=0  strideFrom=1  copyTo=Output port  copyToAddressSource=Specify via dialog  copyToAddress=hex2dec('00002000')  copyToSrcCode=myVariableDst  dataTypeTo=uint16  useOffsetTo=off  offsetToSrc=Specify via dialog  offsetTo=0  strideTo=1  sampleTime=-1  useInitValue=off  initValueSrc=Specify constant value  initValue=1  initValueSrcCode=myInitValueVariable  useAsMask=off  maskOperator=bitwise AND  useTermValue=off  termValue=1  isRealtimeEnabled=off  emitCCBeforeWrite=off  CCBeforeWrite=/* Custom Code Before Write*/  emitCCAfterWrite=off  CCAfterWrite=/* Custom Code After Write*/  useDMACopy=off  enableBlockingMode=off
  CAP_value : Outport
  wires:
  CAP1FBOT/1 -> CAP_value/1

== system m20150807_motor28335_21/Scaling/Subsystem/speed_calculator ==
  In1 : Inport
  Add : Sum  Inputs=+-  OutDataTypeStr=uint16
  Data Type Conversion1 : DataTypeConversion  OutDataTypeStr=fixdt(1,32,10)  ConvertRealWorld=Stored Integer (SI)
  Data Type Conversion2 : DataTypeConversion  OutDataTypeStr=int16  ConvertRealWorld=Stored Integer (SI)
  IQN1 to IQN2 : tiiqmathlib/IQN1 to IQN2  New_Q=17
  Rate Transition : RateTransition  Integrity=off  OutPortSampleTime=0.01
  Unit Delay : UnitDelay  SampleTime=-1
  Out1 : Outport
  wires:
  In1/1 -> Rate Transition/1
  Rate Transition/1 -> Add/1, Unit Delay/1
  Unit Delay/1 -> Add/2
  IQN1 to IQN2/1 -> Out1/1
  Add/1 -> Data Type Conversion2/1
  Data Type Conversion1/1 -> IQN1 to IQN2/1
  Data Type Conversion2/1 -> Data Type Conversion1/1

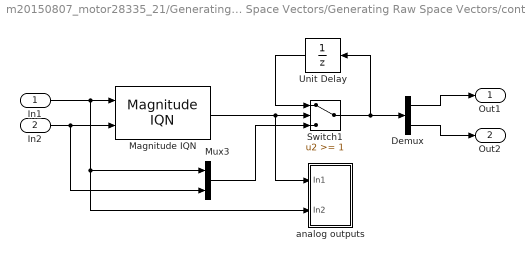
== system m20150807_motor28335_21/Generating Space Vectors/Generating Raw Space Vectors/control/saturation ==
  In1 : Inport
  In2 : Inport  Port=2
  Demux : Demux  Outputs=2
  Magnitude IQN : tiiqmathlib/Magnitude IQN
  Mux3 : Mux  Inputs=2
  Switch1 : Switch  Threshold=1
  Unit Delay : UnitDelay  InitialCondition=[0 0]  SampleTime=-1
  analog outputs : Subsystem
  Out1 : Outport
  Out2 : Outport  Port=2
  wires:
  Magnitude IQN/1 -> Switch1/2, analog outputs/1(In1)
  In1/1 -> Magnitude IQN/1, Mux3/1, analog outputs/2(In2)
  In2/1 -> Magnitude IQN/2, Mux3/2
  Mux3/1 -> Switch1/3
  Switch1/1 -> Unit Delay/1, Demux/1
  Unit Delay/1 -> Switch1/1
  Demux/1 -> Out1/1
  Demux/2 -> Out2/1

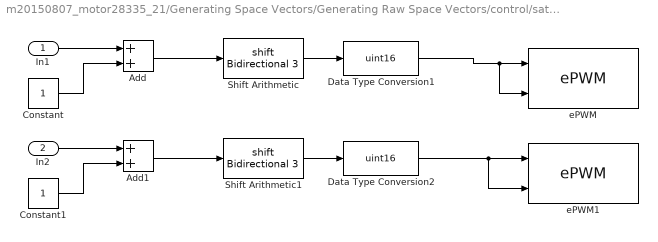
== system m20150807_motor28335_21/Generating Space Vectors/Generating Raw Space Vectors/control/saturation/analog outputs ==
  In1 : Inport
  In2 : Inport  Port=2
  Add : Sum
  Add1 : Sum
  Constant : Constant  OutDataTypeStr=fixdt(1,32,17)
  Constant1 : Constant  OutDataTypeStr=fixdt(1,32,17)
  Data Type Conversion1 : DataTypeConversion  OutDataTypeStr=uint16  ConvertRealWorld=Stored Integer (SI)
  Data Type Conversion2 : DataTypeConversion  OutDataTypeStr=uint16  ConvertRealWorld=Stored Integer (SI)
  Shift Arithmetic : ArithShift  BitShiftNumber=3
  Shift Arithmetic1 : ArithShift  BitShiftNumber=3
  ePWM : c280xlib/ePWM  checkMode=off  useModule=ePWM4  periodUnits=Clock cycles  timerSource=Specify via dialog  timerPeriod_clk=37500  timerPeriod_sec=0.0001  countingMode=Up-Down  synchronizationOption=Disable  synchronizationEnable=off  phaseActiveEnable=Disable  phaseDirection=Count down after sync  phaseActive=0  clockPrescale=1  HSclockPrescale=1  ePWMxAStatus=on  CMPAUnits=Clock cycles  CMPASource=Input port  CMPAValue_per=50  CMPAValue_clk=0  ePWMxAactionLogic1=Do nothing  ePWMxAactionLogic2=Clear  ePWMxAactionLogic3=Set  ePWMxAactionLogic4=Do nothing  ePWMxAactionLogic5=Do nothing  ePWMxAactionLogic6=Do nothing  ePWMxALoadMode=Load on CTR=Zero  ePWMxACSFenable=off  ePWMxACSFvalue=Forcing Disable  ePWMxASFreload=Zero  enHRPWM=off  HRPWM_LoadMode=CTR=ZERO  HRPWM_CTLMode=Phase control mode  HRPWM_EDGMode=Both edge  enSFO=on  ePWMxBStatus=on  CMPBUnits=Clock cycles  CMPBSource=Input port  CMPBValue_per=50  CMPBValue_clk=0  ePWMxBactionLogic1=Do nothing  ePWMxBactionLogic2=Clear  ePWMxBactionLogic3=Do nothing  ePWMxBactionLogic4=Do nothing  ePWMxBactionLogic5=Set  ePWMxBactionLogic6=Do nothing  ePWMxBLoadMode=Load on CTR=Zero  ePWMxBCSFenable=off  ePWMxBCSFvalue=Forcing Disable  ePWMxBSFreload=Zero  enableDBePWMxA=on  enableDBePWMxB=on  DBpolarity=AH  DBedgeDelay=Positive  DBSource_ePWMxA=ePWMxA  DBSource_ePWMxB=ePWMxA  DBperiodSource=Specify via dialog  REDperiod=15  FEDperiod=15  adcstartModuleA=off  adcrequestEventA=First event  adcstartEventA=CTR=Zero  adcstartModuleB=off  adcrequestEventB=First event  adcstartEventB=CTR=Zero  intEn=off  intPrd=First event  intSel=CTR=Zero  chopperEnable=off  chopperFrequency=1  chopperFirstwidth=1  chopperDuty=12.5%  tripZonesource=Specify via dialog  tzselOSHT1=off  tzselOSHT2=off  tzselOSHT3=off  tzselOSHT4=off  tzselOSHT5=off  tzselOSHT6=off  tzselCBC1=off  tzselCBC2=off  tzselCBC3=off  tzselCBC4=off  tzselCBC5=off  tzselCBC6=off  enTzOstIntr=off  enTzCbcIntr=off  ePWMxAforced=No action  ePWMxBforced=No action  timerPeriod=-1  ePWMxAValue=0  ePWMxBValue=0  tripZoneoption=OSHT
  ePWM1 : c280xlib/ePWM  checkMode=off  useModule=ePWM5  periodUnits=Clock cycles  timerSource=Specify via dialog  timerPeriod_clk=37500  timerPeriod_sec=0.0001  countingMode=Up-Down  synchronizationOption=Disable  synchronizationEnable=off  phaseActiveEnable=Disable  phaseDirection=Count down after sync  phaseActive=0  clockPrescale=1  HSclockPrescale=1  ePWMxAStatus=on  CMPAUnits=Clock cycles  CMPASource=Input port  CMPAValue_per=50  CMPAValue_clk=0  ePWMxAactionLogic1=Do nothing  ePWMxAactionLogic2=Clear  ePWMxAactionLogic3=Set  ePWMxAactionLogic4=Do nothing  ePWMxAactionLogic5=Do nothing  ePWMxAactionLogic6=Do nothing  ePWMxALoadMode=Load on CTR=Zero  ePWMxACSFenable=off  ePWMxACSFvalue=Forcing Disable  ePWMxASFreload=Zero  enHRPWM=off  HRPWM_LoadMode=CTR=ZERO  HRPWM_CTLMode=Phase control mode  HRPWM_EDGMode=Both edge  enSFO=on  ePWMxBStatus=on  CMPBUnits=Clock cycles  CMPBSource=Input port  CMPBValue_per=50  CMPBValue_clk=0  ePWMxBactionLogic1=Do nothing  ePWMxBactionLogic2=Clear  ePWMxBactionLogic3=Do nothing  ePWMxBactionLogic4=Do nothing  ePWMxBactionLogic5=Set  ePWMxBactionLogic6=Do nothing  ePWMxBLoadMode=Load on CTR=Zero  ePWMxBCSFenable=off  ePWMxBCSFvalue=Forcing Disable  ePWMxBSFreload=Zero  enableDBePWMxA=on  enableDBePWMxB=on  DBpolarity=AH  DBedgeDelay=Positive  DBSource_ePWMxA=ePWMxA  DBSource_ePWMxB=ePWMxA  DBperiodSource=Specify via dialog  REDperiod=15  FEDperiod=15  adcstartModuleA=off  adcrequestEventA=First event  adcstartEventA=CTR=Zero  adcstartModuleB=off  adcrequestEventB=First event  adcstartEventB=CTR=Zero  intEn=off  intPrd=First event  intSel=CTR=Zero  chopperEnable=off  chopperFrequency=1  chopperFirstwidth=1  chopperDuty=12.5%  tripZonesource=Specify via dialog  tzselOSHT1=off  tzselOSHT2=off  tzselOSHT3=off  tzselOSHT4=off  tzselOSHT5=off  tzselOSHT6=off  tzselCBC1=off  tzselCBC2=off  tzselCBC3=off  tzselCBC4=off  tzselCBC5=off  tzselCBC6=off  enTzOstIntr=off  enTzCbcIntr=off  ePWMxAforced=No action  ePWMxBforced=No action  timerPeriod=-1  ePWMxAValue=0  ePWMxBValue=0  tripZoneoption=OSHT
  wires:
  In1/1 -> Add/1
  Constant/1 -> Add/2
  Add/1 -> Shift Arithmetic/1
  Shift Arithmetic/1 -> Data Type Conversion1/1
  Data Type Conversion1/1 -> ePWM/2, ePWM/1
  In2/1 -> Add1/1
  Constant1/1 -> Add1/2
  Add1/1 -> Shift Arithmetic1/1
  Shift Arithmetic1/1 -> Data Type Conversion2/1
  Data Type Conversion2/1 -> ePWM1/2, ePWM1/1
